simulink model "step14"  (R2016b)
settings: Solver=VariableStepAuto  StartTime=0.0  StopTime=30  RelTol=1e-3
values from neighbouring files (symbols this model uses):
  ACL = A - B*gainK    [EE547FinalProject.m]
  B = [0;B1;0;B2]    [EE547FinalProject.m]
  C = [1 0 0 0; 0 1 0 0; 0 0 1 0; 0 0 0 1]    [EE547FinalProject.m]
  D = zeros(size(C,1),size(B,2))    [EE547FinalProject.m]
  xini = [0 0 0 0]    [EE547FinalProject.m]
settings Model: Creator=muller  LastModifiedBy=muller

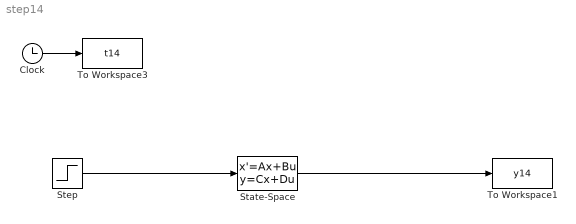
== system step14 ==
  Clock : Clock
  State-Space : StateSpace  A=ACL  B=B  C=C  D=D  X0=xini
  Step : Step  SampleTime=0
  To Workspace1 : ToWorkspace  VariableName=y14  SampleTime=-1
  To Workspace3 : ToWorkspace  VariableName=t14  SampleTime=-1
  wires:
  Clock/1 -> To Workspace3/1
  State-Space/1 -> To Workspace1/1
  Step/1 -> State-Space/1
